simulink model "ex2"  (R2021a)
settings: Solver=VariableStepAuto  StartTime=0.0  StopTime=10.0  RelTol=1e-3
settings Model: Creator=lenovo  LastModifiedBy=lenovo

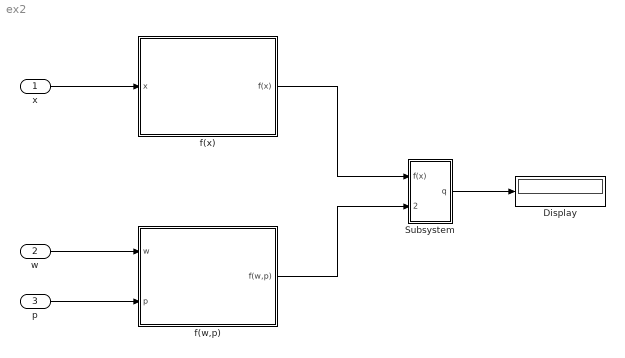
== system ex2 ==
  x : Inport
  w : Inport  Port=2
  p : Inport  Port=3
  Display : Display
  Subsystem : Subsystem
  f(w,p) : Subsystem
  f(x) : Subsystem
  wires:
  x/1 -> f(x)/1(x)
  w/1 -> f(w,p)/1(w)
  p/1 -> f(w,p)/2(p)
  f(x)/1(f(x)) -> Subsystem/1(f(x))
  f(w,p)/1(f(w,p)) -> Subsystem/2(f(w,p))
  Subsystem/1(q) -> Display/1

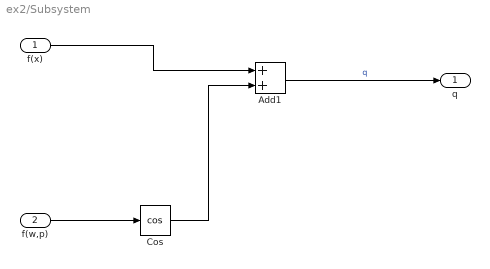
== system ex2/Subsystem ==
  f(x) : Inport
  f(w,p) : Inport  Port=2
  Add1 : Sum
  Cos : Trigonometry  Operator=cos
  q : Outport
  wires:
  Cos/1 -> Add1/2
  f(x)/1 -> Add1/1
  Add1/1 -> q/1  "q"
  f(w,p)/1 -> Cos/1

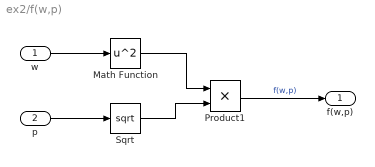
== system ex2/f(w,p) ==
  w : Inport
  p : Inport  Port=2
  Math Function : Math  Operator=square  SaturateOnIntegerOverflow=on
  Product1 : Product
  Sqrt : Sqrt  SaturateOnIntegerOverflow=on
  f(w,p) : Outport
  wires:
  Sqrt/1 -> Product1/2
  Product1/1 -> f(w,p)/1  "f(w,p)"
  Math Function/1 -> Product1/1
  p/1 -> Sqrt/1
  w/1 -> Math Function/1

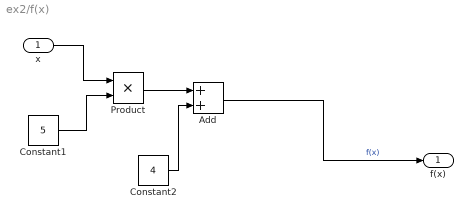
== system ex2/f(x) ==
  x : Inport
  Add : Sum
  Constant1 : Constant  Value=5
  Constant2 : Constant  Value=4
  Product : Product
  f(x) : Outport
  wires:
  Add/1 -> f(x)/1  "f(x)"
  Constant2/1 -> Add/2
  x/1 -> Product/1
  Product/1 -> Add/1
  Constant1/1 -> Product/2
